simulink model "Exercise10"  (Simulink 7.2)
settings: Solver=ode45  StartTime=0.0  StopTime=10.0  RelTol=1e-3
undefined symbols (not defined in the file): des_figposition, des_subsystemblock, des_subsysteminport, des_subsystemoutport, des_subsystemsupportblock
libraries: simeventstranslate1 x2, simeventsqueue1 x2, simeventsgenerators1 x2, simeventsrouting1 x1, simeventssink1 x1, simeventsserver1 x1
settings Model: Creator=Inderjot  LastModifiedBy=Inderjot
settings SimEventsCC: propLogEventsScheduled=0  propLogEventsExecuted=0  propLogDepartureEvents=0  propDisplayEventCalendar=0  propDiagAttribOutput=1  propDiagFcnCallOutput=1  propDiagStatOutput=0

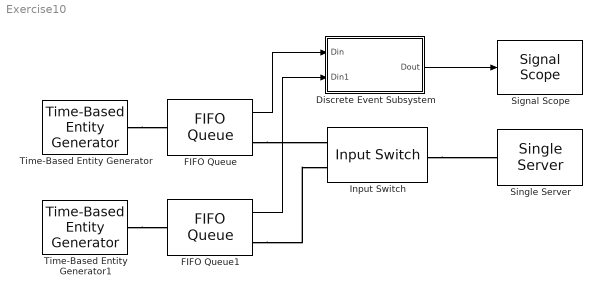
== system Exercise10 ==
  Discrete Event Subsystem : Subsystem  LoadFcn=des_subsystemblock(gcb, 'load');  InitFcn=des_subsystemblock(gcb, 'init');  StartFcn=des_subsystemblock(gcb, 'start');  StopFcn=des_subsystemblock(gcb, 'stop');
      settings: CopyFcn=des_subsystemblock(gcb, 'copy');  DeleteFcn=des_subsystemblock(gcb, 'delete');  UndoDeleteFcn=des_subsystemblock(gcb, 'undodelete');  ModelCloseFcn=des_subsystemblock(gcb, 'modelclose');  PreSaveFcn=des_subsystemblock(gcb, 'presave');  NameChangeFcn=des_subsystemblock(gcb, 'namechange');  OpenFcn=des_subsystemblock(gcb, 'open');  ParentCloseFcn=des_subsystemblock(gcb, 'parentclose');  ErrorFcn=des_subsystemerror
      mask Type: Discrete Event Subsystem
      mask Help: helpview(simeventsbhelp);
  FIFO Queue : simeventsqueue1/FIFO Queue  Priority=1  SystemSampleTime=-1  Capacity=25  EnableTOPort=off  StatNumberDeparted=Off  StatNumberInBlock=On  StatPendingEntity=Off  StatAverageWait=Off  StatAverageQueueLength=Off  StatNumberTimedout=Off
  FIFO Queue1 : simeventsqueue1/FIFO Queue  Priority=1  SystemSampleTime=-1  Capacity=25  EnableTOPort=off  StatNumberDeparted=Off  StatNumberInBlock=On  StatPendingEntity=Off  StatAverageWait=Off  StatAverageQueueLength=Off  StatNumberTimedout=Off
  Input Switch : simeventsrouting1/Input Switch  Priority=1  SystemSampleTime=-1  NumberInputPorts=2  SwitchingCriterion=Round robin  InitialSeed=23453  SpecifyEventPriority=off  PriorityInputSwitchSelectPort=4000  StatNumberDeparted=Off  StatLastArrivalPort=Off  EvaluatedNumPorts=2
  Signal Scope : simeventssink1/Signal Scope  Priority=1  SystemSampleTime=-1  PlotType=Stair  InputType=Signal  NumInputs=1  AttributeNameY=Count  XInputOptionSignal=Event time  XInputOptionEntity=Event time  AttributeNameX=Count  EnableEntityOutport=on  XMin=0  XMax=10  XLimitExceededOption=Stretch axis limits  YLimitExceededOption=Stretch axis limits  AxisGrid=on  AxisLegend=off  LineDisables=""  LineColors=b  LineStyles=-  LineMarkers=.  OpenScopeAtSimStart=on  Title=""  YLabel=""  XLabel=Time  FigurePosition=des_figposition([5 60 25 25])  AxisZoom=off  DataStoreOption=Limited  DataPointsLimit=10000  StatNumberArrived=Off  ShowCountPlotted=off  ShowToolbar=on
      settings: YMin=0  YMax=10
  Single Server : simeventsserver1/Single Server  Priority=1  SystemSampleTime=-1  ServiceTimeFrom=Dialog  ServiceTime=1  AttributeName=ServiceTime  PriorityServiceCompletion=500  PermitPreemption=off  SortingAttributeName=PriorityAttributeName  SortingDirection=Ascending  WriteToAttribute=off  ResidualAttributeName=ResidualServiceTime  CreateAttribute=on  EnableTOPort=off  StatNumberDeparted=Off  StatNumberInBlock=Off  StatNumberPreempted=Off  StatPendingEntity=Off  StatAverageWait=Off  StatUtilization=Off  StatNumberTimedout=Off
  Time-Based Entity Generator : simeventsgenerators1/Entity Generators/Time-Based Entity Generator  Priority=1  DialogController=des_ddg_create  DialogControllerArgs=DataTag15  SystemSampleTime=-1  GenerateEntitiesUpon=Intergeneration time from dialog  Distribution=Constant  Minimum=0  Maximum=1  Mean=1  InitialSeed=12345  Period=1  PriorityEntityGeneration=300  GenerateEntityAtSimulationStart=on  ResponseWhenBlocked=Pause generation  ResponseWhenUnblocked=Immediate restart  EntityType=Blank  StatNumberDeparted=Off  StatPendingEntity=Off  StatAverageIntergenerationTime=Off
  Time-Based Entity Generator1 : simeventsgenerators1/Entity Generators/Time-Based Entity Generator  Priority=1  DialogController=des_ddg_create  DialogControllerArgs=DataTag17  SystemSampleTime=-1  GenerateEntitiesUpon=Intergeneration time from dialog  Distribution=Constant  Minimum=0  Maximum=1  Mean=1  InitialSeed=12345  Period=1  PriorityEntityGeneration=300  GenerateEntityAtSimulationStart=on  ResponseWhenBlocked=Pause generation  ResponseWhenUnblocked=Immediate restart  EntityType=Blank  StatNumberDeparted=Off  StatPendingEntity=Off  StatAverageIntergenerationTime=Off
  wires:
  FIFO Queue/1 -> Discrete Event Subsystem/1(Din)
  FIFO Queue1/1 -> Discrete Event Subsystem/2(Din1)
  Discrete Event Subsystem/1(Dout) -> Signal Scope/1
  connections:
  FIFO Queue/RConn1 -- Input Switch/LConn1
  FIFO Queue1/RConn1 -- Input Switch/LConn2
  Input Switch/RConn1 -- Single Server/LConn1
  Time-Based Entity Generator/RConn1 -- FIFO Queue/LConn1
  Time-Based Entity Generator1/RConn1 -- FIFO Queue1/LConn1

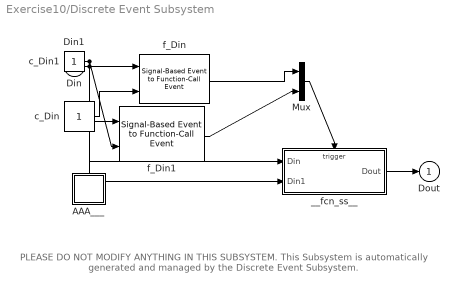
== system Exercise10/Discrete Event Subsystem ==
  note: PLEASE DO NOT MODIFY ANYTHING IN THIS SUBSYSTEM.
      | This Subsystem is automatically generated and
      | managed by the Discrete Event Subsystem.
  Din : Inport  DataType=double  OutDataType=sfix(16)  OutScaling=2^0  OutDataTypeStr=double
  Din1 : Inport  Port=2  DataType=double  OutDataTypeStr=double
  AAA___ : Subsystem  LoadFcn=des_subsystemsupportblock(gcb, 'load');  InitFcn=des_subsystemsupportblock(gcb, 'init');  StartFcn=des_subsystemsupportblock(gcb, 'start');  StopFcn=des_subsystemsupportblock(gcb, 'stop');
      settings: CopyFcn=des_subsystemsupportblock(gcb, 'copy');  DeleteFcn=des_subsystemsupportblock(gcb, 'delete');  UndoDeleteFcn=des_subsystemsupportblock(gcb, 'undodelete');  ModelCloseFcn=des_subsystemsupportblock(gcb, 'modelclose');  PreSaveFcn=des_subsystemsupportblock(gcb, 'presave');  NameChangeFcn=des_subsystemsupportblock(gcb, 'namechange');  OpenFcn=des_subsystemsupportblock(gcb, 'open');  ParentCloseFcn=des_subsystemsupportblock(gcb, 'parentclose');
  Mux : Mux  Inputs=2
  __fcn_ss__ : Subsystem  TreatAsAtomicUnit=on
      settings: PropExecContextOutsideSubsystem=on
  c_Din : Constant  OutDataType=sfix(16)  OutScaling=2^0
  c_Din1 : Constant
  f_Din : simeventstranslate1/Signal-Based Event to Function-Call Event  Priority=1  SystemSampleTime=-1  GenerateFunctionCallUpon=Sample time hit from port ts  SignalEdgeOption=Rising  EnableE1Port=on  EnableF2Port=off  EnableE2Port=off  SpecifyEventPriority=off  PriorityFunctionCall=20  FunctionCallDelayFrom=Dialog  DelayFunctionCall=0  StatNumberF1Calls=Off  StatNumberF2Calls=Off  MaskBlockType=DESS_EVENT_PORT
  f_Din1 : simeventstranslate1/Signal-Based Event to Function-Call Event  Priority=1  SystemSampleTime=-1  GenerateFunctionCallUpon=Sample time hit from port ts  SignalEdgeOption=Rising  EnableE1Port=on  EnableF2Port=off  EnableE2Port=off  SpecifyEventPriority=off  PriorityFunctionCall=20  FunctionCallDelayFrom=Dialog  DelayFunctionCall=0  StatNumberF1Calls=Off  StatNumberF2Calls=Off  MaskBlockType=DESS_EVENT_PORT
  Dout : Outport  OutDataType=sfix(16)  OutScaling=2^0
  wires:
  __fcn_ss__/1(Dout) -> Dout/1
  f_Din/1 -> Mux/1
  c_Din/1 -> f_Din/2
  Mux/1 -> __fcn_ss__/Trigger
  f_Din1/1 -> Mux/2
  c_Din1/1 -> f_Din1/2
  Din/1 -> f_Din/1, __fcn_ss__/1(Din)
  Din1/1 -> f_Din1/1, __fcn_ss__/2(Din1)

== system Exercise10/Discrete Event Subsystem/AAA___ ==

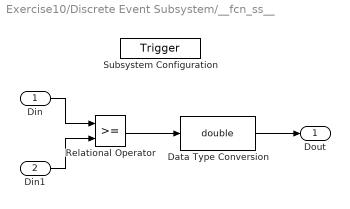
== system Exercise10/Discrete Event Subsystem/__fcn_ss__ ==
  Din : Inport  LoadFcn=des_subsysteminport(gcb, 'load');  InitFcn=des_subsysteminport(gcb, 'init');  StartFcn=des_subsysteminport(gcb, 'start');  StopFcn=des_subsysteminport(gcb, 'stop');  OutDataType=sfix(16)  OutScaling=2^0  mask(Discrete Event Inport){PermitSubsystemEvents=on, TypeOfEvent=Sample time hit, SignalEdgeOption=Rising, SpecifyEventPriority=off, PrioritySubsystemEvent=20}
      mask prompts: PermitSubsystemEvents "Execute subsystem upon signal-based events"; TypeOfEvent "Type of signal-based event:"; SignalEdgeOption "Type of change in signal value:"; SpecifyEventPriority "Resolve simultaneous signal updates according to event priority"; PrioritySubsystemEvent "Event priority:"
      mask help: Input port for a Discrete Event Subsystem block. This block can conditionally execute the subsystem upon signal-based events that meet specified criteria.
      mask init:
      | des_subsystemmask(gcb, 'init','apply')
      settings: CopyFcn=des_subsysteminport(gcb, 'copy');  DeleteFcn=des_subsysteminport(gcb, 'delete');  UndoDeleteFcn=des_subsysteminport(gcb, 'undodelete');  ModelCloseFcn=des_subsysteminport(gcb, 'modelclose');  PreSaveFcn=des_subsysteminport(gcb, 'presave');  NameChangeFcn=des_subsysteminport(gcb, 'namechange');  ParentCloseFcn=des_subsysteminport(gcb, 'parentclose');
      mask Help: helpview(simeventsbhelp);
      mask StyleString: checkbox,popup(Change in signal|Trigger|Sample time hit),popup(Rising|Falling|Either),checkbox,edit
      mask CallbackString: des_subsystemmask(gcb, 'cbPermitSubsystemEvents', 'noapply');|des_subsystemmask(gcb,'cbTypeOfEvent','noapply');||des_subsystemmask(gcb, 'cbSpecifyEventPriority', 'noapply');|
  Din1 : Inport  LoadFcn=des_subsysteminport(gcb, 'load');  InitFcn=des_subsysteminport(gcb, 'init');  StartFcn=des_subsysteminport(gcb, 'start');  StopFcn=des_subsysteminport(gcb, 'stop');  Port=2  OutDataType=sfix(16)  OutScaling=2^0  mask(Discrete Event Inport){PermitSubsystemEvents=on, TypeOfEvent=Sample time hit, SignalEdgeOption=Rising, SpecifyEventPriority=off, PrioritySubsystemEvent=20}
      mask prompts: PermitSubsystemEvents "Execute subsystem upon signal-based events"; TypeOfEvent "Type of signal-based event:"; SignalEdgeOption "Type of change in signal value:"; SpecifyEventPriority "Resolve simultaneous signal updates according to event priority"; PrioritySubsystemEvent "Event priority:"
      mask help: Input port for a Discrete Event Subsystem block. This block can conditionally execute the subsystem upon signal-based events that meet specified criteria.
      mask init:
      | des_subsystemmask(gcb, 'init','apply')
      settings: CopyFcn=des_subsysteminport(gcb, 'copy');  DeleteFcn=des_subsysteminport(gcb, 'delete');  UndoDeleteFcn=des_subsysteminport(gcb, 'undodelete');  ModelCloseFcn=des_subsysteminport(gcb, 'modelclose');  PreSaveFcn=des_subsysteminport(gcb, 'presave');  NameChangeFcn=des_subsysteminport(gcb, 'namechange');  ParentCloseFcn=des_subsysteminport(gcb, 'parentclose');
      mask Help: helpview(simeventsbhelp);
      mask StyleString: checkbox,popup(Change in signal|Trigger|Sample time hit),popup(Rising|Falling|Either),checkbox,edit
      mask CallbackString: des_subsystemmask(gcb, 'cbPermitSubsystemEvents', 'noapply');|des_subsystemmask(gcb,'cbTypeOfEvent','noapply');||des_subsystemmask(gcb, 'cbSpecifyEventPriority', 'noapply');|
  Subsystem Configuration : TriggerPort  TriggerType=function-call
      settings: CopyFcn=des_subsystemconfigblock(gcb, 'copy');  DeleteFcn=des_subsystemconfigblock(gcb, 'delete');  UndoDeleteFcn=des_subsystemconfigblock(gcb, 'undodelete');
      mask Type: Subsystem Configuration
      mask Description: Configuration for a Discrete Event Subsystem block. Every discrete event subsystem window must contain exactly one copy of this configuration block. Do not delete this block.
      mask Help: helpview(simeventsbhelp);
      mask Display: disp('Do Not Delete');
  Data Type Conversion : DataTypeConversion  OutDataTypeMode=double  OutDataType=sfix(16)  OutScaling=2^0  OutDataTypeStr=double
  Relational Operator : RelationalOperator  LogicOutDataTypeMode=boolean  OutDataTypeStr=boolean
  Dout : Outport  LoadFcn=des_subsystemoutport(gcb, 'load');  InitFcn=des_subsystemoutport(gcb, 'init');  StartFcn=des_subsystemoutport(gcb, 'start');  StopFcn=des_subsystemoutport(gcb, 'stop');  OutDataType=sfix(16)  OutScaling=2^0
      settings: CopyFcn=des_subsystemoutport(gcb, 'copy');  DeleteFcn=des_subsystemoutport(gcb, 'delete');  UndoDeleteFcn=des_subsystemoutport(gcb, 'undodelete');  ModelCloseFcn=des_subsystemoutport(gcb, 'modelclose');  PreSaveFcn=des_subsystemoutport(gcb, 'presave');  NameChangeFcn=des_subsystemoutport(gcb, 'namechange');  ParentCloseFcn=des_subsystemoutport(gcb, 'parentclose');
      mask Type: Discrete Event Outport
      mask Description: Provide an output port for a Discrete Event Subsystem block.
      mask Help: helpview(simeventsbhelp);
  wires:
  Din/1 -> Relational Operator/1
  Din1/1 -> Relational Operator/2
  Relational Operator/1 -> Data Type Conversion/1
  Data Type Conversion/1 -> Dout/1
